simulink model "BPSK"  (R2018a)
settings: Solver=VariableStepAuto  StartTime=0.0  StopTime=10.0  RelTol=1e-3
libraries: dspmathops x2, dspsrcs4 x2, commrandsrc3 x1
settings Model: Creator=Subhankar  LastModifiedBy=Souhardhya Paul

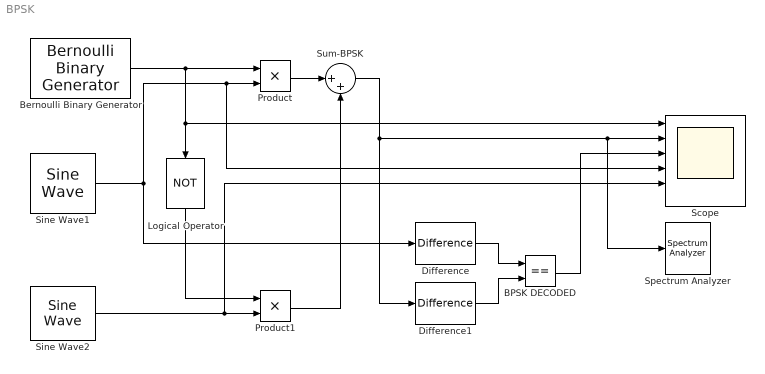
== system BPSK ==
  BPSK DECODED : RelationalOperator  Operator===  OutDataTypeStr=boolean  RndMeth=Simplest
  Bernoulli Binary Generator : commrandsrc3/Bernoulli Binary Generator  ProbabilityOfZero=0.5  SeedSource=Parameter  Seed=61  SampleTime=0.1  SamplesPerFrame=1  OutputDataType=double  SimulateUsing=Interpreted execution
  Difference : dspmathops/Difference  Run=Yes  dim=Columns  Dimension=1  roundingMode=Floor  overflowMode=off  outputDataTypeStr=Inherit: Same as accumulator  outputMin=[]  outputMax=[]  outputLastDataTypeStr=Inherit: Same as accumulator
      settings: SourceProductName=DSP System Toolbox  SourceProductBaseCode=DS
  Difference1 : dspmathops/Difference  Run=Yes  dim=Columns  Dimension=1  roundingMode=Floor  overflowMode=off  outputDataTypeStr=Inherit: Same as accumulator  outputMin=[]  outputMax=[]  outputLastDataTypeStr=Inherit: Same as accumulator
      settings: SourceProductName=DSP System Toolbox  SourceProductBaseCode=DS
  Logical Operator : Logic  Operator=NOT  AllPortsSameDT=off  OutDataTypeStr=boolean
  Product : Product
  Product1 : Product
  Scope : Scope  NumInputPorts=6
  Sine Wave1 : dspsrcs4/Sine Wave  Amplitude=1  Frequency=100  Phase=0  SampleMode=Discrete  OutComplex=Real  CompMethod=Trigonometric fcn  TableSize=Speed  SampleTime=1/1000  SamplesPerFrame=1  ResetState=Restart at time zero  OutputFrames=off  dataType=double  wordLen=16  udDataType=sfix(16)  fracBitsMode=Best precision  numFracBits=15  OutDataTypeStr=double  LastOutDataTypeStr=double
  Sine Wave2 : dspsrcs4/Sine Wave  Amplitude=1  Frequency=100  Phase=pi  SampleMode=Discrete  OutComplex=Real  CompMethod=Trigonometric fcn  TableSize=Speed  SampleTime=1/1000  SamplesPerFrame=1  ResetState=Restart at time zero  OutputFrames=off  dataType=double  wordLen=16  udDataType=sfix(16)  fracBitsMode=Best precision  numFracBits=15  OutDataTypeStr=double  LastOutDataTypeStr=double
  Spectrum Analyzer : SpectrumAnalyzer
  Sum-BPSK : Sum  Inputs=|++
  wires:
  Bernoulli Binary Generator/1 -> Logical Operator/1, Scope/1, Product/1
  Logical Operator/1 -> Product1/1
  Sine Wave2/1 -> Scope/5, Product1/2
  Product/1 -> Sum-BPSK/1
  Product1/1 -> Sum-BPSK/2
  Sum-BPSK/1 -> Difference1/1, Scope/2, Spectrum Analyzer/1
  Difference/1 -> BPSK DECODED/1
  Difference1/1 -> BPSK DECODED/2
  BPSK DECODED/1 -> Scope/3
  Sine Wave1/1 -> Difference/1, Scope/4, Product/2
